simulink library "aerolibprivatev1p5"  (Simulink 5.0)
values from neighbouring files (symbols this model uses):
  s = aeroliblist    [asbhelp.m]
undefined symbols (not defined in the file or in its folder): F, kg, m, MIL
libraries: aerolibconvert x5, aerolibwind2 x3, aerolib6dof2 x2, aerolib3dof2 x1, aerolibatmos2 x1
settings Model: Creator=sgage  LastModifiedBy=sgage  ExtModeAutoUpdateStatusClock=off  TargetHWChar=2  TargetHWWordLengths=8,16,32,32

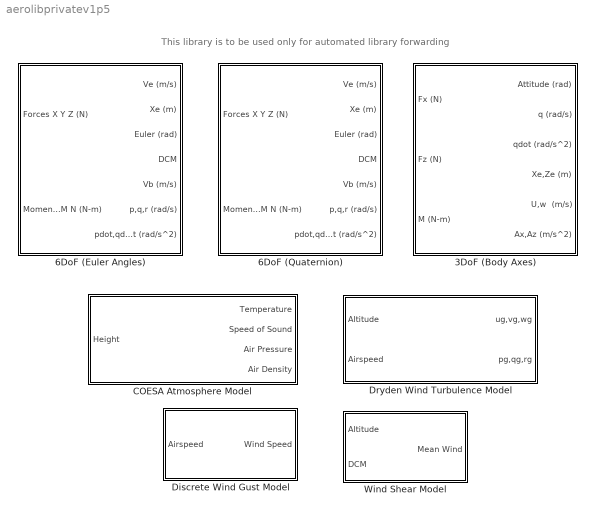
== system aerolibprivatev1p5 ==
  note: This library is to be used only for automated library forwarding
  3DoF (Body Axes) : Subsystem  mask(3DOF bridge){v_ini=100, theta_ini=0, alpha_ini=0, q_ini=0, pos_ini=[0 0], mass=1.0, Iyy=1.0, g=9.81}
      mask prompts: v_ini "Initial velocity (m/s):"; theta_ini "Initial body attitude (rad):"; alpha_ini "Initial incidence (rad):"; q_ini "Initial body rotation rate (rad/s):"; pos_ini "Initial position (m):"; mass "Mass (kg):"; Iyy "Inertia (kg.m^2):"; g "Acceleration due to gravity [m/s/s]:"
      mask help:
      | Block to bridge changes from version 1.0 and 1.0.1 to version 1.5.  Please consider updating your model.
      |
      | Integrate the three-degrees-of-freedom equations of motion to determine body position, velocity, attitude, and related values.
      mask Help: web(asbhelp('3dofbodyaxes'));
      mask Display:
      | port_label('input',1,'F_{X} (N)','texmode','on');
      | port_label('input',2,'F_{Z} (N)','texmode','on');
      | port_label('input',3,'M (N-m)','texmode','on');
      | port_label('output',1,'\theta (rad)','texmode','on');
      | port_label('output',2,'\omega_{Y} (rad/s)','texmode','on');
      | port_label('output',3,'d\omega_{Y}/dt','texmode','on');
      | port_label('output',5,'U w (m/s)','texmode','on');
      | port_label('output',4,'X_e Z_e (m)','texmode','on');
      | port_label('output',6,'A_X A_Z','texmode','on');
  6DoF (Euler Angles) : Subsystem  mask(6DOF EA Bridge){xme_0=[0 0 0], Vm_0=[0 0 0], eul_0=[ 0 0 0], pm_0=[0 0 0], Mass=1.0, Inertia=eye(3)}
      mask prompts: xme_0 "Initial position in inertial axes [Xe,Ye,Ze] (m):"; Vm_0 "Initial velocity in body axes [U,v,w] (m/s):"; eul_0 "Initial Euler orientation [roll, pitch, yaw] (rad):"; pm_0 "Initial body rotation rates [p,q,r] (rad/s):"; Mass "Mass (kg):"; Inertia "Inertia matrix (kg.m^2):"
      mask help:
      | Block to bridge changes from version 1.0 and 1.0.1 to version 1.5.  Please consider updating your model.
      |
      | Integrate the six-degrees-of-freedom equations of motion using an Euler angle representation for the orientation of the body in space.
      mask Help: web(asbhelp('6dofeulerangles'));
      mask Display:
      | port_label('input',1,'F_{XYZ} (N)','texmode','on');
      | port_label('input',2,'M_{XYZ} (N-m)','texmode','on');
      | port_label('output',1,'V_e (m/s)','texmode','on');
      | port_label('output',2,'X_e (m)','texmode','on');
      | port_label('output',3,'\phi \theta \psi (rad)','texmode','on');
      | port_label('output',4,'DCM','texmode','on');
      | port_label('output',5,'V_b (m/s)','texmode','on');
      | port_label('output',6,'\omega (rad/s)','texmode','on');
      | port_label('output',7,'d\omega/dt','texmode','on');
      | disp('Euler Angles')
  6DoF (Quaternion) : Subsystem  mask(6DOF Q Bridge){xme_0=[0 0 0], Vm_0=[0 0 0], eul_0=[ 0 0 0], pm_0=[0 0 0], Mass=1.0, Inertia=eye(3), k_quat=1.0}
      mask prompts: xme_0 "Initial position in inertial axes [Xe,Ye,Ze] (m):"; Vm_0 "Initial velocity in body axes [U,v,w] (m/s):"; eul_0 "Initial Euler orientation [roll, pitch, yaw] (rad):"; pm_0 "Initial body rotation rates [p,q,r] (rad/s):"; Mass "Mass (kg):"; Inertia "Inertia matrix (kg.m^2):"; k_quat "Gain for quaternion normalization:"
      mask help:
      | Block to bridge changes from version 1.0 and 1.0.1 to version 1.5.  Please consider updating your model.
      |
      | Integrate the six-degrees-of-freedom equations of motion using a quaternion representation for the orientation of the body in space.
      mask Help: web(asbhelp('6dofquaternion'));
      mask Display:
      | port_label('input',1,'F_{XYZ} (N)','texmode','on');
      | port_label('input',2,'M_{XYZ} (N-m)','texmode','on');
      | port_label('output',1,'V_e (m/s)','texmode','on');
      | port_label('output',2,'X_e (m)','texmode','on');
      | port_label('output',3,'\phi \theta \psi (rad)','texmode','on');
      | port_label('output',4,'DCM','texmode','on');
      | port_label('output',5,'V_b (m/s)','texmode','on');
      | port_label('output',6,'\omega (rad/s)','texmode','on');
      | port_label('output',7,'d\omega/dt','texmode','on');
      | disp('Quaternion')
  COESA Atmosphere Model : Subsystem  mask(COESA Atmosphere Bridge){units=Metric}
      mask help:
      | Block to bridge changes from version 1.0 and 1.0.1 to version 1.5.  Please consider updating your model.
      |
      | Calculate 1976 COESA-extended U.S. Standard Atmosphere. Given geopotential altitude, calculate absolute temperature, pressure, and density using standard interpolation formulas (linear in temperature and logarithmic in pressure).
      |
      | Extrapolate temperature linearly and pressure  logarithmically beyond the range
      |            0 <= altitude <= 84852 m
      |
      | Density is calculated using a perfect gas relationship.
      |
      | Data used is from the 15-OCT-1976 COESA extensions to the U.S. Standard Atmosphere, 1976, published by the U.S. Government Printing Office, Washington, D.C.
      |
      | The unit system selected applies to both input and outputs.
      mask init:
      | [ports] = aeroicon('aeroblkcoesa','icon');
      mask Help: web(asbhelp('COESA Atmosphere Model'));
      mask StyleString: popup(Metric|English)
      mask Display:
      | port_label(ports(1).type,ports(1).port,ports(1).txt);
      | port_label(ports(2).type,ports(2).port,ports(2).txt);
      | port_label(ports(3).type,ports(3).port,ports(3).txt);
      | port_label(ports(4).type,ports(4).port,ports(4).txt);
      | port_label(ports(5).type,ports(5).port,ports(5).txt);
  Discrete Wind Gust Model : Subsystem  mask(Discrete Wind Gust Bridge){v_units=meters/second, Gx=on, Gy=on, Gz=on, t_0=5, d_m=[120 120 80], v_m=[3.5 3.5 3.0]}
      mask prompts: v_units "Units of velocity:"; Gx "Check for gust in u-axis"; Gy "Check for gust in v-axis"; Gz "Check for gust in w-axis"; t_0 "Gust start time (seconds):"; d_m "Gust length [dx dy dz] (meters):"; v_m "Gust amplitude [ug vg wg] (meters/second):"
      mask help:
      | Block to bridge changes from version 1.0 and 1.0.1 to version 1.5.  Please consider updating your model.
      |
      | Generate a discrete wind gust. The gust profile takes the '1-cosine' form.
      mask init:
      | blk = gcb;
      | blk_g = [blk, '/Discrete Wind Gust Model'];
      | if strcmp(v_units, 'meters/second')
      |   mask_text1='m';
      |   mask_text2='m/s';
      |   set_param(blk_g,'units','Metric (MKS)');
      | elseif strcmp(v_units, 'feet/second')
      |   mask_text1='ft';
      |   mask_text2='ft/s';
      |   set_param(blk_g,'units','English (Velocity in ft/s)');
      | else
      |   mask_text1='ft';
      |   mask_text2='knots';
      |   set_param(blk_g,'units','English (Velocity in kts)');
      | end
      | if (Gx == 1)
      | 	set_param(blk_g,'Gx','on');
      | else
      | 	set_param(blk_g,'Gx','off');
      | end
      | if (Gy == 1)
      | 	set_param(blk_g,'Gy','on');
      | else
      | 	set_param(blk_g,'Gy','off');
      | end
      | if (Gz == 1)
      | 	set_param(blk_g,'Gz','on');
      | else
      | 	set_param(blk_g,'Gz','off');
      | end
      mask Help: web(asbhelp('discretewindgustmodel'));
      mask StyleString: popup(meters/second|feet/second|knots),checkbox,checkbox,checkbox,edit,edit,edit
      mask CallbackString: aeroicon('aeroblkwindgust')||||||
      mask Display:
      | port_label('output', 1, ['V_{wind} (', mask_text2, ')'],'texmode','on')
      | port_label('input', 1, ['V (', mask_text2, ')'],'texmode','on')
  Dryden Wind Turbulence Model : Subsystem  mask(Dryden Wind Turbulence Bridge){v_units=meters/second, W20=15, TurbProb=10^-1, L_high=533, Wingspan=10, ts=0.1, Seed=[23341 23342 23343 23344], T_on=on}
      mask prompts: v_units "Units of velocity:"; W20 "Wind speed at 6 m defines the low-altitude intensity (meters/second):"; TurbProb "Probability of exceedance of high-altitude intensity"; L_high "Scale length at medium/high altitudes (meters):"; Wingspan "Wingspan (meters):"; ts "Band-limited noise sample time (seconds):"; Seed "Noise seeds [ug vg wg pg]:"; T_on "Turbulence on"
      mask help:
      | Block to bridge changes from version 1.0 and 1.0.1 to version 1.5.  Please consider updating your model.
      |
      | Generate atmospheric turbulence. White noise is passed through a filter to give the turbulence the Dryden velocity spectra.
      mask init:
      | blk=gcb;
      | blk_t=[blk '/Dryden Wind Turbulence Model'];
      | if strcmp(v_units, 'meters/second')
      |     mask_text1='m';
      |     mask_text2='m/s';
      |     set_param(blk_t,'units','Metric (MKS)');
      | elseif strcmp(v_units, 'feet/second')
      |     mask_text1='ft';
      |     mask_text2='ft/s';
      |     set_param(blk_t,'units','English (Velocity in ft/s)');
      | else
      |     mask_text1='ft';
      |     mask_text2='knots';
      |     set_param(blk_t,'units','English (Velocity in kts)');
      | end
      | if T_on == 1
      |   set_param(blk_t,'T_on','on');
      | else
      |   set_param(blk_t,'T_on','off');
      | end
      | if strcmp(TurbProb,'2x10^-1')
      |     set_param(blk_t,'TurbProb','2x10^-1');
      | elseif strcmp(TurbProb,'10^-1')
      |     set_param(blk_t,'TurbProb','10^-1');
      | elseif strcmp(TurbProb,'10^-2 - Light ')
      |     set_param(blk_t,'TurbProb','10^-2 - Light ');
      | elseif strcmp(TurbProb,'10^-3 - Moderate')
      | 	set_param(blk_t,'TurbProb','10^-3 - Moderate');
      | elseif strcmp(TurbProb,'10^-4')
      |     set_param(blk_t,'TurbProb','10^-4');
      | elseif strcmp(TurbProb,'10^-5 - Severe')
      | 	set_param(blk_t,'TurbProb','10^-5 - Severe');
      | else
      |     set_param(blk_t,'TurbProb','10^-6');
      | end
      mask Help: web(asbhelp('Dryden Wind Turbulence Model (Continuous)'));
      mask StyleString: popup(meters/second|feet/second|knots),edit,popup(2x10^-1|10^-1|10^-2 - Light |10^-3 - Moderate|10^-4|10^-5 - Severe|10^-6),edit,edit,edit,edit,checkbox
      mask CallbackString: aeroicon('aeroblkwindturb')|||||||
      mask Display:
      | port_label('output', 1, ['V_{wind} (', mask_text2, ')'],'texmode','on')
      | port_label('output', 2, '\omega_{wind} (rad/sec)','texmode','on')
      | port_label('input', 1, ['h (', mask_text1, ')'])
      | port_label('input', 2, ['V (', mask_text2, ')'])
  Wind Shear Model : Subsystem  mask(Wind Shear Bridge){v_units=meters/second, phase=Category C - Terminal Flight Phase, W_20=15, Wdeg=0}
      mask prompts: v_units "Units of velocity:"; phase "Flight phase:"; W_20 "Wind speed at 6 meters altitude (meters/second):"; Wdeg "Wind direction at 6 meters altitude (degrees clockwise from north):"
      mask help:
      | Block to bridge changes from version 1.0 and 1.0.1 to version 1.5.  Please consider updating your model.
      |
      | Calculate the wind shear from conditions measured at a height of 6 meters (20 feet) above the ground.
      mask init:
      | blk=gcb;
      | blk_s=[blk '/Wind Shear Model'];
      | if strcmp(v_units, 'meters/second')
      |   mask_text1='m';
      |   mask_text2='m/s';
      |   set_param(blk_s,'units','Metric (MKS)');
      | elseif strcmp(v_units, 'feet/second')
      |   mask_text1='ft';
      |   mask_text2='ft/s';
      |   set_param(blk_s,'units','English (Velocity in ft/s)');
      | else
      |   mask_text1='ft';
      |   mask_text2='knots';
      |   set_param(blk_s,'units','English (Velocity in kts)');
      | end
      | if phase == 1
      |   set_param(blk_s,'phase','Category C - Terminal Flight Phase');
      | else
      |   set_param(blk_s,'phase','Other');
      | end
      mask Help: web(asbhelp('windshearmodel'));
      mask StyleString: popup(meters/second|feet/second|knots),popup(Category C - Terminal Flight Phase|Other),edit,edit
      mask CallbackString: aeroicon('aeroblkwindshear')|||
      mask Display:
      | port_label('output', 1, ['V_{wind} (', mask_text2, ')'],'texmode','on')
      | port_label('input', 1, ['h (', mask_text1, ')'])
      | port_label('input', 2, 'DCM')

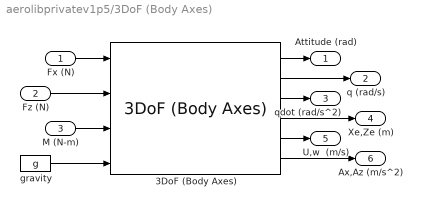
== system aerolibprivatev1p5/3DoF (Body Axes) ==
  Fx (N) : Inport  ShowAdditionalParam=on  DataType=double
  Fz (N) : Inport  Port=2  ShowAdditionalParam=on  DataType=double
  M (N-m) : Inport  Port=3  ShowAdditionalParam=on  DataType=double
  3DoF (Body Axes) : aerolib3dof2/3DoF (Body Axes)  units=Metric (MKS)  mtype=Fixed  v_ini=v_ini  theta_ini=theta_ini  alpha_ini=alpha_ini  q_ini=q_ini  pos_ini=pos_ini  mass=mass  mass_e=0.5  mass_f=3.0  Iyy=Iyy  Iyy_e=0.5  Iyy_f=3.0  g_in=External  g=9.81
  gravity : Constant  Value=g
  Attitude (rad) : Outport  InitialOutput=0
  q (rad/s) : Outport  Port=2  InitialOutput=0
  qdot (rad/s^2) : Outport  Port=3  InitialOutput=0
  Xe,Ze (m) : Outport  Port=4  InitialOutput=0
  "U,w  (m/s) " : Outport  Port=5  InitialOutput=0
  Ax,Az (m/s^2) : Outport  Port=6  InitialOutput=0
  wires:
  gravity/1 -> 3DoF (Body Axes)/4
  M (N-m)/1 -> 3DoF (Body Axes)/3
  Fz (N)/1 -> 3DoF (Body Axes)/2
  Fx (N)/1 -> 3DoF (Body Axes)/1
  3DoF (Body Axes)/1 -> Attitude (rad)/1
  3DoF (Body Axes)/2 -> q (rad/s)/1
  3DoF (Body Axes)/3 -> qdot (rad/s^2)/1
  3DoF (Body Axes)/4 -> Xe,Ze (m)/1
  3DoF (Body Axes)/5 -> "U,w  (m/s) "/1
  3DoF (Body Axes)/6 -> Ax,Az (m/s^2)/1

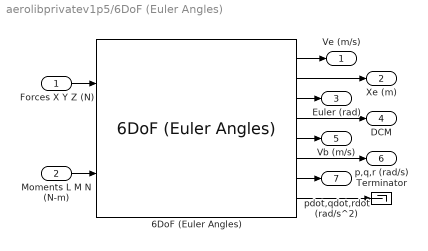
== system aerolibprivatev1p5/6DoF (Euler Angles) ==
  Forces X Y Z (N) : Inport  ShowAdditionalParam=on  DataType=double
  Moments L M N (N-m) : Inport  Port=2  ShowAdditionalParam=on  DataType=double
  6DoF (Euler Angles) : aerolib6dof2/6DoF (Euler Angles)  units=Metric (MKS)  mtype=Fixed  rep=Euler Angles  xme_0=xme_0  Vm_0=Vm_0  eul_0=eul_0  pm_0=pm_0  mass_0=Mass  mass_e=0.5  mass_f=2.0  inertia=Inertia  inertia_e=eye(3)  inertia_f=2*eye(3)  k_quat=1.0
  Terminator : Terminator
  Ve (m/s) : Outport
  Xe (m) : Outport  Port=2
  Euler (rad) : Outport  Port=3
  DCM : Outport  Port=4
  Vb (m/s) : Outport  Port=5
  p,q,r (rad/s) : Outport  Port=6
  pdot,qdot,rdot (rad/s^2) : Outport  Port=7
  wires:
  6DoF (Euler Angles)/7 -> pdot,qdot,rdot (rad/s^2)/1
  Moments L M N (N-m)/1 -> 6DoF (Euler Angles)/2
  6DoF (Euler Angles)/6 -> p,q,r (rad/s)/1
  6DoF (Euler Angles)/5 -> Vb (m/s)/1
  6DoF (Euler Angles)/4 -> DCM/1
  6DoF (Euler Angles)/3 -> Euler (rad)/1
  Forces X Y Z (N)/1 -> 6DoF (Euler Angles)/1
  6DoF (Euler Angles)/2 -> Xe (m)/1
  6DoF (Euler Angles)/1 -> Ve (m/s)/1
  6DoF (Euler Angles)/8 -> Terminator/1

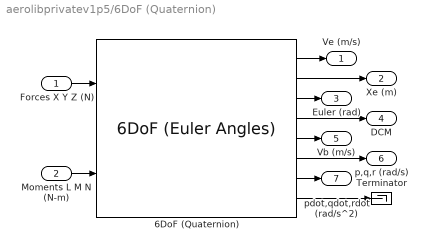
== system aerolibprivatev1p5/6DoF (Quaternion) ==
  Forces X Y Z (N) : Inport  ShowAdditionalParam=on  DataType=double
  Moments L M N (N-m) : Inport  Port=2  ShowAdditionalParam=on  DataType=double
  6DoF (Quaternion) : aerolib6dof2/6DoF (Euler Angles)  units=Metric (MKS)  mtype=Fixed  rep=Quaternion  xme_0=xme_0  Vm_0=Vm_0  eul_0=eul_0  pm_0=pm_0  mass_0=Mass  mass_e=0.5  mass_f=2.0  inertia=Inertia  inertia_e=eye(3)  inertia_f=2*eye(3)  k_quat=k_quat
  Terminator : Terminator
  Ve (m/s) : Outport
  Xe (m) : Outport  Port=2
  Euler (rad) : Outport  Port=3
  DCM : Outport  Port=4
  Vb (m/s) : Outport  Port=5
  p,q,r (rad/s) : Outport  Port=6
  pdot,qdot,rdot (rad/s^2) : Outport  Port=7
  wires:
  6DoF (Quaternion)/7 -> pdot,qdot,rdot (rad/s^2)/1
  Moments L M N (N-m)/1 -> 6DoF (Quaternion)/2
  6DoF (Quaternion)/6 -> p,q,r (rad/s)/1
  6DoF (Quaternion)/5 -> Vb (m/s)/1
  6DoF (Quaternion)/4 -> DCM/1
  6DoF (Quaternion)/3 -> Euler (rad)/1
  Forces X Y Z (N)/1 -> 6DoF (Quaternion)/1
  6DoF (Quaternion)/2 -> Xe (m)/1
  6DoF (Quaternion)/1 -> Ve (m/s)/1
  6DoF (Quaternion)/8 -> Terminator/1

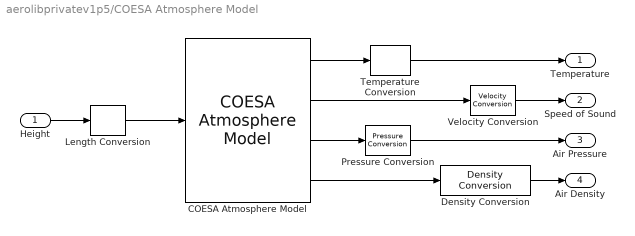
== system aerolibprivatev1p5/COESA Atmosphere Model ==
  Height : Inport
  COESA Atmosphere Model : aerolibatmos2/COESA Atmosphere Model  units=Metric (MKS)  spec=1976 COESA-extended U.S. Standard Atmosphere  model=Profile  profile_var=High temperature  profile_percent=1%  profile_alt=5 km (16404 ft)  envelope_var=High temperature  envelope_percent=1%  action=Warning
  Density Conversion : aerolibconvert/Density Conversion  IU=kg/m^3  OU=kg/m^3
  Length Conversion : aerolibconvert/Length Conversion  IU=m  OU=m
  Pressure Conversion : aerolibconvert/Pressure Conversion  IU=Pa  OU=Pa
  Temperature Conversion : aerolibconvert/Temperature Conversion  IU=K  OU=K
  Velocity Conversion : aerolibconvert/Velocity Conversion  IU=m/s  OU=m/s
  Temperature : Outport
  Speed of Sound : Outport  Port=2
  Air Pressure : Outport  Port=3
  Air Density : Outport  Port=4
  wires:
  Length Conversion/1 -> COESA Atmosphere Model/1
  Velocity Conversion/1 -> Speed of Sound/1
  COESA Atmosphere Model/2 -> Velocity Conversion/1
  COESA Atmosphere Model/1 -> Temperature Conversion/1
  COESA Atmosphere Model/3 -> Pressure Conversion/1
  COESA Atmosphere Model/4 -> Density Conversion/1
  Temperature Conversion/1 -> Temperature/1
  Height/1 -> Length Conversion/1
  Pressure Conversion/1 -> Air Pressure/1
  Density Conversion/1 -> Air Density/1

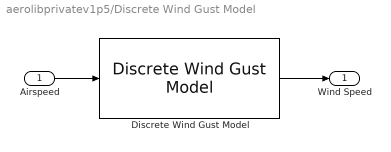
== system aerolibprivatev1p5/Discrete Wind Gust Model ==
  Airspeed : Inport
  Discrete Wind Gust Model : aerolibwind2/Discrete Wind Gust Model  units=Metric (MKS)  Gx=on  Gy=on  Gz=on  t_0=t_0  d_m=d_m  v_m=v_m
  Wind Speed : Outport
  wires:
  Discrete Wind Gust Model/1 -> Wind Speed/1
  Airspeed/1 -> Discrete Wind Gust Model/1

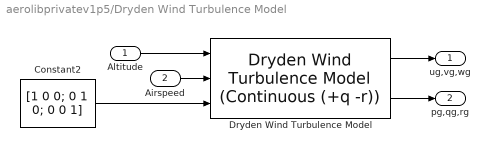
== system aerolibprivatev1p5/Dryden Wind Turbulence Model ==
  Altitude : Inport
  Airspeed : Inport  Port=2
  Constant2 : Constant  Value=[1 0 0; 0 1 0; 0 0 1]
  Dryden Wind Turbulence Model : aerolibwind2/Dryden Wind Turbulence Model  (Continuous (+q -r))  units=Metric (MKS)  spec=MIL-F-8785C  model=Continuous Dryden (+q -r)  W20=W20  Wdeg=0  TurbProb=10^-1  L_high=L_high  Wingspan=Wingspan  ts=ts  Seed=Seed  T_on=on
  ug,vg,wg : Outport
  pg,qg,rg : Outport  Port=2
  wires:
  Altitude/1 -> Dryden Wind Turbulence Model/1
  Airspeed/1 -> Dryden Wind Turbulence Model/2
  Dryden Wind Turbulence Model/1 -> ug,vg,wg/1
  Dryden Wind Turbulence Model/2 -> pg,qg,rg/1
  Constant2/1 -> Dryden Wind Turbulence Model/3

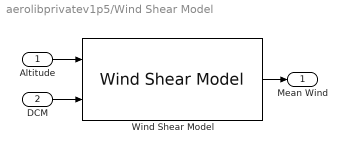
== system aerolibprivatev1p5/Wind Shear Model ==
  Altitude : Inport
  DCM : Inport  Port=2
  Wind Shear Model : aerolibwind2/Wind Shear Model  units=Metric (MKS)  phase=Category C - Terminal Flight Phase  W_20=W_20  Wdeg=Wdeg
  Mean Wind : Outport
  wires:
  Wind Shear Model/1 -> Mean Wind/1
  Altitude/1 -> Wind Shear Model/1
  DCM/1 -> Wind Shear Model/2
